simulink model "sei"  (Simulink 6.2)
settings: Solver=ode45  StartTime=0.0  StopTime=10.0  RelTol=1e-3
libraries: dsparch4 x287, cdsEpicsOut x108, cdsEpicsIn x18, cdsRms x18, Matrix8x x15, cdsSwitch1 x12, cdsProduct x9, Matrix88 x9, cdsSwitch x6, cdsSubtract8 x3, cdsRampSwitch x3, cdsSWD1 x3
(part 2 of 6)

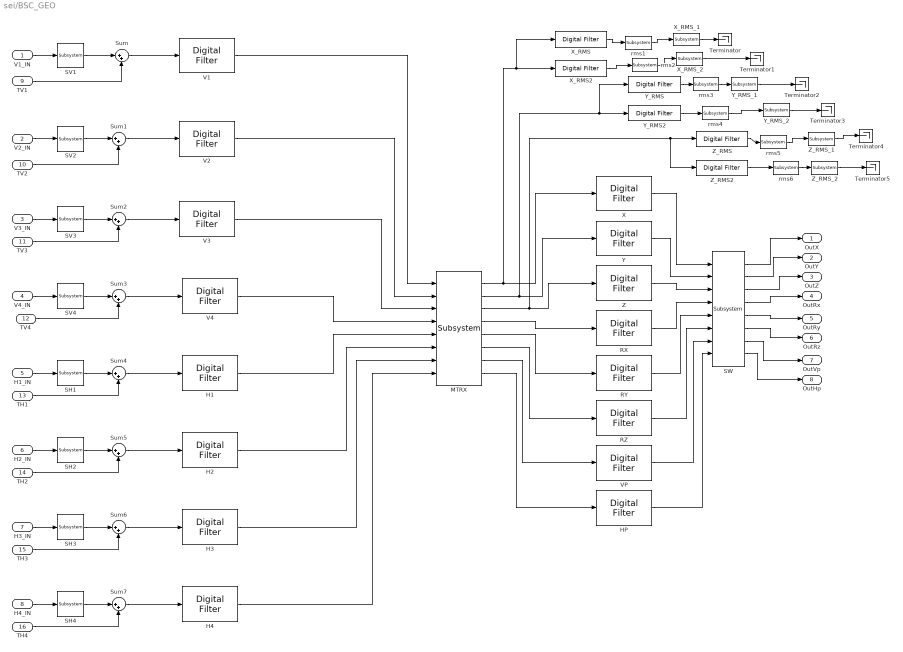
== system sei/BSC_GEO ==
  V1_IN : Inport  Port=1  LatchInput=off
  V2_IN : Inport  Port=2  LatchInput=off
  V3_IN : Inport  Port=3  LatchInput=off
  V4_IN : Inport  Port=4  LatchInput=off
  H1_IN : Inport  Port=5  LatchInput=off
  H2_IN : Inport  Port=6  LatchInput=off
  H3_IN : Inport  Port=7  LatchInput=off
  H4_IN : Inport  Port=8  LatchInput=off
  TV1 : Inport  Port=9  LatchInput=off
  TV2 : Inport  Port=10  LatchInput=off
  TV3 : Inport  Port=11  LatchInput=off
  TV4 : Inport  Port=12  LatchInput=off
  TH1 : Inport  Port=13  LatchInput=off
  TH2 : Inport  Port=14  LatchInput=off
  TH3 : Inport  Port=15  LatchInput=off
  TH4 : Inport  Port=16  LatchInput=off
  H1 : dsparch4/Digital Filter  DialogController=dspDDGCreate  DialogControllerArgs=DataTag26  TypePopup=IIR (poles & zeros)  IIRFiltStruct=Direct form II transposed  AllPoleFiltStruct=Direct form  FIRFiltStruct=Direct form  CoeffSource=Specify via dialog  NumCoeffs=[1 2]  DenCoeffs=[1 0.1]  BiQuadCoeffs=[1 0.3 0.4 1 0.1 0.2]  LatticeCoeffs=[0.2 0.4]  denIgnore=on  FiltPerSampPopup=One filter per frame  IC=0  ICnum=0  ICden=0  roundingMode=Floor  overflowMode=off  ScaleValues=1  scaleValueFracLength=14  stageInFracLength=15  stageOutFracLength=15
  H2 : dsparch4/Digital Filter  DialogController=dspDDGCreate  DialogControllerArgs=DataTag27  TypePopup=IIR (poles & zeros)  IIRFiltStruct=Direct form II transposed  AllPoleFiltStruct=Direct form  FIRFiltStruct=Direct form  CoeffSource=Specify via dialog  NumCoeffs=[1 2]  DenCoeffs=[1 0.1]  BiQuadCoeffs=[1 0.3 0.4 1 0.1 0.2]  LatticeCoeffs=[0.2 0.4]  denIgnore=on  FiltPerSampPopup=One filter per frame  IC=0  ICnum=0  ICden=0  roundingMode=Floor  overflowMode=off  ScaleValues=1  scaleValueFracLength=14  stageInFracLength=15  stageOutFracLength=15
  H3 : dsparch4/Digital Filter  DialogController=dspDDGCreate  DialogControllerArgs=DataTag28  TypePopup=IIR (poles & zeros)  IIRFiltStruct=Direct form II transposed  AllPoleFiltStruct=Direct form  FIRFiltStruct=Direct form  CoeffSource=Specify via dialog  NumCoeffs=[1 2]  DenCoeffs=[1 0.1]  BiQuadCoeffs=[1 0.3 0.4 1 0.1 0.2]  LatticeCoeffs=[0.2 0.4]  denIgnore=on  FiltPerSampPopup=One filter per frame  IC=0  ICnum=0  ICden=0  roundingMode=Floor  overflowMode=off  ScaleValues=1  scaleValueFracLength=14  stageInFracLength=15  stageOutFracLength=15
  H4 : dsparch4/Digital Filter  DialogController=dspDDGCreate  DialogControllerArgs=DataTag29  TypePopup=IIR (poles & zeros)  IIRFiltStruct=Direct form II transposed  AllPoleFiltStruct=Direct form  FIRFiltStruct=Direct form  CoeffSource=Specify via dialog  NumCoeffs=[1 2]  DenCoeffs=[1 0.1]  BiQuadCoeffs=[1 0.3 0.4 1 0.1 0.2]  LatticeCoeffs=[0.2 0.4]  denIgnore=on  FiltPerSampPopup=One filter per frame  IC=0  ICnum=0  ICden=0  roundingMode=Floor  overflowMode=off  ScaleValues=1  scaleValueFracLength=14  stageInFracLength=15  stageOutFracLength=15
  HP : dsparch4/Digital Filter  DialogController=dspDDGCreate  DialogControllerArgs=DataTag30  TypePopup=IIR (poles & zeros)  IIRFiltStruct=Direct form II transposed  AllPoleFiltStruct=Direct form  FIRFiltStruct=Direct form  CoeffSource=Specify via dialog  NumCoeffs=[1 2]  DenCoeffs=[1 0.1]  BiQuadCoeffs=[1 0.3 0.4 1 0.1 0.2]  LatticeCoeffs=[0.2 0.4]  denIgnore=on  FiltPerSampPopup=One filter per frame  IC=0  ICnum=0  ICden=0  roundingMode=Floor  overflowMode=off  ScaleValues=1  scaleValueFracLength=14  stageInFracLength=15  stageOutFracLength=15
  MTRX : Matrix8x/Subsystem
  RX : dsparch4/Digital Filter  DialogController=dspDDGCreate  DialogControllerArgs=DataTag31  TypePopup=IIR (poles & zeros)  IIRFiltStruct=Direct form II transposed  AllPoleFiltStruct=Direct form  FIRFiltStruct=Direct form  CoeffSource=Specify via dialog  NumCoeffs=[1 2]  DenCoeffs=[1 0.1]  BiQuadCoeffs=[1 0.3 0.4 1 0.1 0.2]  LatticeCoeffs=[0.2 0.4]  denIgnore=on  FiltPerSampPopup=One filter per frame  IC=0  ICnum=0  ICden=0  roundingMode=Floor  overflowMode=off  ScaleValues=1  scaleValueFracLength=14  stageInFracLength=15  stageOutFracLength=15
  RY : dsparch4/Digital Filter  DialogController=dspDDGCreate  DialogControllerArgs=DataTag32  TypePopup=IIR (poles & zeros)  IIRFiltStruct=Direct form II transposed  AllPoleFiltStruct=Direct form  FIRFiltStruct=Direct form  CoeffSource=Specify via dialog  NumCoeffs=[1 2]  DenCoeffs=[1 0.1]  BiQuadCoeffs=[1 0.3 0.4 1 0.1 0.2]  LatticeCoeffs=[0.2 0.4]  denIgnore=on  FiltPerSampPopup=One filter per frame  IC=0  ICnum=0  ICden=0  roundingMode=Floor  overflowMode=off  ScaleValues=1  scaleValueFracLength=14  stageInFracLength=15  stageOutFracLength=15
  RZ : dsparch4/Digital Filter  DialogController=dspDDGCreate  DialogControllerArgs=DataTag33  TypePopup=IIR (poles & zeros)  IIRFiltStruct=Direct form II transposed  AllPoleFiltStruct=Direct form  FIRFiltStruct=Direct form  CoeffSource=Specify via dialog  NumCoeffs=[1 2]  DenCoeffs=[1 0.1]  BiQuadCoeffs=[1 0.3 0.4 1 0.1 0.2]  LatticeCoeffs=[0.2 0.4]  denIgnore=on  FiltPerSampPopup=One filter per frame  IC=0  ICnum=0  ICden=0  roundingMode=Floor  overflowMode=off  ScaleValues=1  scaleValueFracLength=14  stageInFracLength=15  stageOutFracLength=15
  SH{1..4} (4 alike) : cdsEpicsOut/Subsystem
  SV{1..4} (4 alike) : cdsEpicsOut/Subsystem
  SW : cdsSwitch/Subsystem
  Sum{,1..7} (8 alike) : Sum  Inputs=|++
  Terminator{,1..5} (6 alike) : Terminator
  V1 : dsparch4/Digital Filter  DialogController=dspDDGCreate  DialogControllerArgs=DataTag34  TypePopup=IIR (poles & zeros)  IIRFiltStruct=Direct form II transposed  AllPoleFiltStruct=Direct form  FIRFiltStruct=Direct form  CoeffSource=Specify via dialog  NumCoeffs=[1 2]  DenCoeffs=[1 0.1]  BiQuadCoeffs=[1 0.3 0.4 1 0.1 0.2]  LatticeCoeffs=[0.2 0.4]  denIgnore=on  FiltPerSampPopup=One filter per frame  IC=0  ICnum=0  ICden=0  roundingMode=Floor  overflowMode=off  ScaleValues=1  scaleValueFracLength=14  stageInFracLength=15  stageOutFracLength=15
  V2 : dsparch4/Digital Filter  DialogController=dspDDGCreate  DialogControllerArgs=DataTag35  TypePopup=IIR (poles & zeros)  IIRFiltStruct=Direct form II transposed  AllPoleFiltStruct=Direct form  FIRFiltStruct=Direct form  CoeffSource=Specify via dialog  NumCoeffs=[1 2]  DenCoeffs=[1 0.1]  BiQuadCoeffs=[1 0.3 0.4 1 0.1 0.2]  LatticeCoeffs=[0.2 0.4]  denIgnore=on  FiltPerSampPopup=One filter per frame  IC=0  ICnum=0  ICden=0  roundingMode=Floor  overflowMode=off  ScaleValues=1  scaleValueFracLength=14  stageInFracLength=15  stageOutFracLength=15
  V3 : dsparch4/Digital Filter  DialogController=dspDDGCreate  DialogControllerArgs=DataTag36  TypePopup=IIR (poles & zeros)  IIRFiltStruct=Direct form II transposed  AllPoleFiltStruct=Direct form  FIRFiltStruct=Direct form  CoeffSource=Specify via dialog  NumCoeffs=[1 2]  DenCoeffs=[1 0.1]  BiQuadCoeffs=[1 0.3 0.4 1 0.1 0.2]  LatticeCoeffs=[0.2 0.4]  denIgnore=on  FiltPerSampPopup=One filter per frame  IC=0  ICnum=0  ICden=0  roundingMode=Floor  overflowMode=off  ScaleValues=1  scaleValueFracLength=14  stageInFracLength=15  stageOutFracLength=15
  V4 : dsparch4/Digital Filter  DialogController=dspDDGCreate  DialogControllerArgs=DataTag37  TypePopup=IIR (poles & zeros)  IIRFiltStruct=Direct form II transposed  AllPoleFiltStruct=Direct form  FIRFiltStruct=Direct form  CoeffSource=Specify via dialog  NumCoeffs=[1 2]  DenCoeffs=[1 0.1]  BiQuadCoeffs=[1 0.3 0.4 1 0.1 0.2]  LatticeCoeffs=[0.2 0.4]  denIgnore=on  FiltPerSampPopup=One filter per frame  IC=0  ICnum=0  ICden=0  roundingMode=Floor  overflowMode=off  ScaleValues=1  scaleValueFracLength=14  stageInFracLength=15  stageOutFracLength=15
  VP : dsparch4/Digital Filter  DialogController=dspDDGCreate  DialogControllerArgs=DataTag38  TypePopup=IIR (poles & zeros)  IIRFiltStruct=Direct form II transposed  AllPoleFiltStruct=Direct form  FIRFiltStruct=Direct form  CoeffSource=Specify via dialog  NumCoeffs=[1 2]  DenCoeffs=[1 0.1]  BiQuadCoeffs=[1 0.3 0.4 1 0.1 0.2]  LatticeCoeffs=[0.2 0.4]  denIgnore=on  FiltPerSampPopup=One filter per frame  IC=0  ICnum=0  ICden=0  roundingMode=Floor  overflowMode=off  ScaleValues=1  scaleValueFracLength=14  stageInFracLength=15  stageOutFracLength=15
  X : dsparch4/Digital Filter  DialogController=dspDDGCreate  DialogControllerArgs=DataTag39  TypePopup=IIR (poles & zeros)  IIRFiltStruct=Direct form II transposed  AllPoleFiltStruct=Direct form  FIRFiltStruct=Direct form  CoeffSource=Specify via dialog  NumCoeffs=[1 2]  DenCoeffs=[1 0.1]  BiQuadCoeffs=[1 0.3 0.4 1 0.1 0.2]  LatticeCoeffs=[0.2 0.4]  denIgnore=on  FiltPerSampPopup=One filter per frame  IC=0  ICnum=0  ICden=0  roundingMode=Floor  overflowMode=off  ScaleValues=1  scaleValueFracLength=14  stageInFracLength=15  stageOutFracLength=15
  X_RMS : dsparch4/Digital Filter  DialogController=dspDDGCreate  DialogControllerArgs=DataTag40  TypePopup=IIR (poles & zeros)  IIRFiltStruct=Direct form II transposed  AllPoleFiltStruct=Direct form  FIRFiltStruct=Direct form  CoeffSource=Specify via dialog  NumCoeffs=[1 2]  DenCoeffs=[1 0.1]  BiQuadCoeffs=[1 0.3 0.4 1 0.1 0.2]  LatticeCoeffs=[0.2 0.4]  denIgnore=on  FiltPerSampPopup=One filter per frame  IC=0  ICnum=0  ICden=0  roundingMode=Floor  overflowMode=off  ScaleValues=1  scaleValueFracLength=14  stageInFracLength=15  stageOutFracLength=15
  X_RMS2 : dsparch4/Digital Filter  DialogController=dspDDGCreate  DialogControllerArgs=DataTag41  TypePopup=IIR (poles & zeros)  IIRFiltStruct=Direct form II transposed  AllPoleFiltStruct=Direct form  FIRFiltStruct=Direct form  CoeffSource=Specify via dialog  NumCoeffs=[1 2]  DenCoeffs=[1 0.1]  BiQuadCoeffs=[1 0.3 0.4 1 0.1 0.2]  LatticeCoeffs=[0.2 0.4]  denIgnore=on  FiltPerSampPopup=One filter per frame  IC=0  ICnum=0  ICden=0  roundingMode=Floor  overflowMode=off  ScaleValues=1  scaleValueFracLength=14  stageInFracLength=15  stageOutFracLength=15
  X_RMS_1 : cdsEpicsOut/Subsystem
  X_RMS_2 : cdsEpicsOut/Subsystem
  Y : dsparch4/Digital Filter  DialogController=dspDDGCreate  DialogControllerArgs=DataTag42  TypePopup=IIR (poles & zeros)  IIRFiltStruct=Direct form II transposed  AllPoleFiltStruct=Direct form  FIRFiltStruct=Direct form  CoeffSource=Specify via dialog  NumCoeffs=[1 2]  DenCoeffs=[1 0.1]  BiQuadCoeffs=[1 0.3 0.4 1 0.1 0.2]  LatticeCoeffs=[0.2 0.4]  denIgnore=on  FiltPerSampPopup=One filter per frame  IC=0  ICnum=0  ICden=0  roundingMode=Floor  overflowMode=off  ScaleValues=1  scaleValueFracLength=14  stageInFracLength=15  stageOutFracLength=15
  Y_RMS : dsparch4/Digital Filter  DialogController=dspDDGCreate  DialogControllerArgs=DataTag43  TypePopup=IIR (poles & zeros)  IIRFiltStruct=Direct form II transposed  AllPoleFiltStruct=Direct form  FIRFiltStruct=Direct form  CoeffSource=Specify via dialog  NumCoeffs=[1 2]  DenCoeffs=[1 0.1]  BiQuadCoeffs=[1 0.3 0.4 1 0.1 0.2]  LatticeCoeffs=[0.2 0.4]  denIgnore=on  FiltPerSampPopup=One filter per frame  IC=0  ICnum=0  ICden=0  roundingMode=Floor  overflowMode=off  ScaleValues=1  scaleValueFracLength=14  stageInFracLength=15  stageOutFracLength=15
  Y_RMS2 : dsparch4/Digital Filter  DialogController=dspDDGCreate  DialogControllerArgs=DataTag44  TypePopup=IIR (poles & zeros)  IIRFiltStruct=Direct form II transposed  AllPoleFiltStruct=Direct form  FIRFiltStruct=Direct form  CoeffSource=Specify via dialog  NumCoeffs=[1 2]  DenCoeffs=[1 0.1]  BiQuadCoeffs=[1 0.3 0.4 1 0.1 0.2]  LatticeCoeffs=[0.2 0.4]  denIgnore=on  FiltPerSampPopup=One filter per frame  IC=0  ICnum=0  ICden=0  roundingMode=Floor  overflowMode=off  ScaleValues=1  scaleValueFracLength=14  stageInFracLength=15  stageOutFracLength=15
  Y_RMS_1 : cdsEpicsOut/Subsystem
  Y_RMS_2 : cdsEpicsOut/Subsystem
  Z : dsparch4/Digital Filter  DialogController=dspDDGCreate  DialogControllerArgs=DataTag45  TypePopup=IIR (poles & zeros)  IIRFiltStruct=Direct form II transposed  AllPoleFiltStruct=Direct form  FIRFiltStruct=Direct form  CoeffSource=Specify via dialog  NumCoeffs=[1 2]  DenCoeffs=[1 0.1]  BiQuadCoeffs=[1 0.3 0.4 1 0.1 0.2]  LatticeCoeffs=[0.2 0.4]  denIgnore=on  FiltPerSampPopup=One filter per frame  IC=0  ICnum=0  ICden=0  roundingMode=Floor  overflowMode=off  ScaleValues=1  scaleValueFracLength=14  stageInFracLength=15  stageOutFracLength=15
  Z_RMS : dsparch4/Digital Filter  DialogController=dspDDGCreate  DialogControllerArgs=DataTag46  TypePopup=IIR (poles & zeros)  IIRFiltStruct=Direct form II transposed  AllPoleFiltStruct=Direct form  FIRFiltStruct=Direct form  CoeffSource=Specify via dialog  NumCoeffs=[1 2]  DenCoeffs=[1 0.1]  BiQuadCoeffs=[1 0.3 0.4 1 0.1 0.2]  LatticeCoeffs=[0.2 0.4]  denIgnore=on  FiltPerSampPopup=One filter per frame  IC=0  ICnum=0  ICden=0  roundingMode=Floor  overflowMode=off  ScaleValues=1  scaleValueFracLength=14  stageInFracLength=15  stageOutFracLength=15
  Z_RMS2 : dsparch4/Digital Filter  DialogController=dspDDGCreate  DialogControllerArgs=DataTag47  TypePopup=IIR (poles & zeros)  IIRFiltStruct=Direct form II transposed  AllPoleFiltStruct=Direct form  FIRFiltStruct=Direct form  CoeffSource=Specify via dialog  NumCoeffs=[1 2]  DenCoeffs=[1 0.1]  BiQuadCoeffs=[1 0.3 0.4 1 0.1 0.2]  LatticeCoeffs=[0.2 0.4]  denIgnore=on  FiltPerSampPopup=One filter per frame  IC=0  ICnum=0  ICden=0  roundingMode=Floor  overflowMode=off  ScaleValues=1  scaleValueFracLength=14  stageInFracLength=15  stageOutFracLength=15
  Z_RMS_1 : cdsEpicsOut/Subsystem
  Z_RMS_2 : cdsEpicsOut/Subsystem
  rms{1..6} (6 alike) : cdsRms/Subsystem
  OutX : Outport
  OutY : Outport  Port=2
  OutZ : Outport  Port=3
  OutRx : Outport  Port=4
  OutRy : Outport  Port=5
  OutRz : Outport  Port=6
  OutVp : Outport  Port=7
  OutHp : Outport  Port=8
  wires:
  H2_IN/1 -> SH2/1
  H3_IN/1 -> SH3/1
  H4_IN/1 -> SH4/1
  MTRX/1 -> X/1, X_RMS2/1, X_RMS/1
  MTRX/2 -> Y/1, Y_RMS2/1, Y_RMS/1
  MTRX/3 -> Z/1, Z_RMS/1, Z_RMS2/1
  MTRX/6 -> RZ/1
  MTRX/7 -> VP/1
  MTRX/8 -> HP/1
  X/1 -> SW/1
  Y/1 -> SW/2
  Z/1 -> SW/3
  RX/1 -> SW/4
  RY/1 -> SW/5
  RZ/1 -> SW/6
  VP/1 -> SW/7
  HP/1 -> SW/8
  MTRX/4 -> RX/1
  MTRX/5 -> RY/1
  SW/1 -> OutX/1
  SW/2 -> OutY/1
  SW/3 -> OutZ/1
  SW/4 -> OutRx/1
  SW/5 -> OutRy/1
  SW/6 -> OutRz/1
  SW/7 -> OutVp/1
  SW/8 -> OutHp/1
  V1/1 -> MTRX/1
  V2/1 -> MTRX/2
  V3/1 -> MTRX/3
  V4/1 -> MTRX/4
  H1/1 -> MTRX/5
  H2/1 -> MTRX/6
  H3/1 -> MTRX/7
  H4/1 -> MTRX/8
  H1_IN/1 -> SH1/1
  V4_IN/1 -> SV4/1
  V3_IN/1 -> SV3/1
  V2_IN/1 -> SV2/1
  V1_IN/1 -> SV1/1
  SV1/1 -> Sum/1
  SV2/1 -> Sum1/1
  SV3/1 -> Sum2/1
  SV4/1 -> Sum3/1
  SH1/1 -> Sum4/1
  SH2/1 -> Sum5/1
  SH3/1 -> Sum6/1
  SH4/1 -> Sum7/1
  TV1/1 -> Sum/2
  TV2/1 -> Sum1/2
  TV3/1 -> Sum2/2
  TV4/1 -> Sum3/2
  TH1/1 -> Sum4/2
  TH2/1 -> Sum5/2
  TH3/1 -> Sum6/2
  TH4/1 -> Sum7/2
  Sum3/1 -> V4/1
  Sum4/1 -> H1/1
  Sum5/1 -> H2/1
  Sum6/1 -> H3/1
  Sum7/1 -> H4/1
  Sum/1 -> V1/1
  Sum1/1 -> V2/1
  Sum2/1 -> V3/1
  X_RMS_1/1 -> Terminator/1
  X_RMS_2/1 -> Terminator1/1
  Y_RMS_2/1 -> Terminator3/1
  Y_RMS_1/1 -> Terminator2/1
  Z_RMS_1/1 -> Terminator4/1
  Z_RMS_2/1 -> Terminator5/1
  X_RMS2/1 -> rms2/1
  X_RMS/1 -> rms1/1
  rms1/1 -> X_RMS_1/1
  rms2/1 -> X_RMS_2/1
  Y_RMS2/1 -> rms4/1
  Y_RMS/1 -> rms3/1
  rms3/1 -> Y_RMS_1/1
  rms4/1 -> Y_RMS_2/1
  Z_RMS2/1 -> rms6/1
  rms6/1 -> Z_RMS_2/1
  Z_RMS/1 -> rms5/1
  rms5/1 -> Z_RMS_1/1

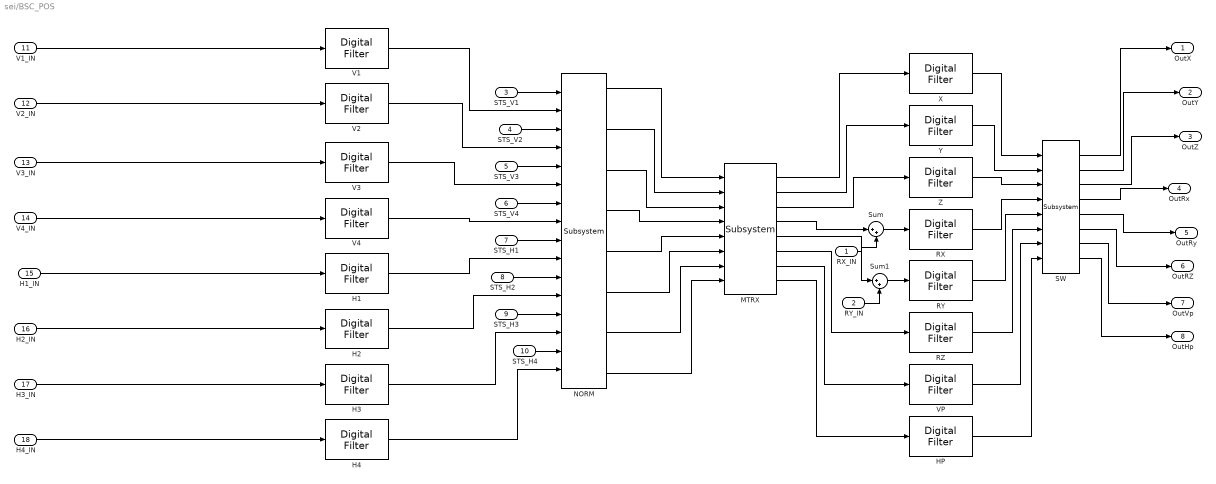
== system sei/BSC_POS ==
  RX_IN : Inport  Port=1  LatchInput=off
  RY_IN : Inport  Port=2  LatchInput=off
  STS_V1 : Inport  Port=3  LatchInput=off
  STS_V2 : Inport  Port=4  LatchInput=off
  STS_V3 : Inport  Port=5  LatchInput=off
  STS_V4 : Inport  Port=6  LatchInput=off
  STS_H1 : Inport  Port=7  LatchInput=off
  STS_H2 : Inport  Port=8  LatchInput=off
  STS_H3 : Inport  Port=9  LatchInput=off
  STS_H4 : Inport  Port=10  LatchInput=off
  V1_IN : Inport  Port=11  LatchInput=off
  V2_IN : Inport  Port=12  LatchInput=off
  V3_IN : Inport  Port=13  LatchInput=off
  V4_IN : Inport  Port=14  LatchInput=off
  H1_IN : Inport  Port=15  LatchInput=off
  H2_IN : Inport  Port=16  LatchInput=off
  H3_IN : Inport  Port=17  LatchInput=off
  H4_IN : Inport  Port=18  LatchInput=off
  H1 : dsparch4/Digital Filter  DialogController=dspDDGCreate  DialogControllerArgs=DataTag48  TypePopup=IIR (poles & zeros)  IIRFiltStruct=Direct form II transposed  AllPoleFiltStruct=Direct form  FIRFiltStruct=Direct form  CoeffSource=Specify via dialog  NumCoeffs=[1 2]  DenCoeffs=[1 0.1]  BiQuadCoeffs=[1 0.3 0.4 1 0.1 0.2]  LatticeCoeffs=[0.2 0.4]  denIgnore=on  FiltPerSampPopup=One filter per frame  IC=0  ICnum=0  ICden=0  roundingMode=Floor  overflowMode=off  ScaleValues=1  scaleValueFracLength=14  stageInFracLength=15  stageOutFracLength=15
  H2 : dsparch4/Digital Filter  DialogController=dspDDGCreate  DialogControllerArgs=DataTag49  TypePopup=IIR (poles & zeros)  IIRFiltStruct=Direct form II transposed  AllPoleFiltStruct=Direct form  FIRFiltStruct=Direct form  CoeffSource=Specify via dialog  NumCoeffs=[1 2]  DenCoeffs=[1 0.1]  BiQuadCoeffs=[1 0.3 0.4 1 0.1 0.2]  LatticeCoeffs=[0.2 0.4]  denIgnore=on  FiltPerSampPopup=One filter per frame  IC=0  ICnum=0  ICden=0  roundingMode=Floor  overflowMode=off  ScaleValues=1  scaleValueFracLength=14  stageInFracLength=15  stageOutFracLength=15
  H3 : dsparch4/Digital Filter  DialogController=dspDDGCreate  DialogControllerArgs=DataTag50  TypePopup=IIR (poles & zeros)  IIRFiltStruct=Direct form II transposed  AllPoleFiltStruct=Direct form  FIRFiltStruct=Direct form  CoeffSource=Specify via dialog  NumCoeffs=[1 2]  DenCoeffs=[1 0.1]  BiQuadCoeffs=[1 0.3 0.4 1 0.1 0.2]  LatticeCoeffs=[0.2 0.4]  denIgnore=on  FiltPerSampPopup=One filter per frame  IC=0  ICnum=0  ICden=0  roundingMode=Floor  overflowMode=off  ScaleValues=1  scaleValueFracLength=14  stageInFracLength=15  stageOutFracLength=15
  H4 : dsparch4/Digital Filter  DialogController=dspDDGCreate  DialogControllerArgs=DataTag51  TypePopup=IIR (poles & zeros)  IIRFiltStruct=Direct form II transposed  AllPoleFiltStruct=Direct form  FIRFiltStruct=Direct form  CoeffSource=Specify via dialog  NumCoeffs=[1 2]  DenCoeffs=[1 0.1]  BiQuadCoeffs=[1 0.3 0.4 1 0.1 0.2]  LatticeCoeffs=[0.2 0.4]  denIgnore=on  FiltPerSampPopup=One filter per frame  IC=0  ICnum=0  ICden=0  roundingMode=Floor  overflowMode=off  ScaleValues=1  scaleValueFracLength=14  stageInFracLength=15  stageOutFracLength=15
  HP : dsparch4/Digital Filter  DialogController=dspDDGCreate  DialogControllerArgs=DataTag52  TypePopup=IIR (poles & zeros)  IIRFiltStruct=Direct form II transposed  AllPoleFiltStruct=Direct form  FIRFiltStruct=Direct form  CoeffSource=Specify via dialog  NumCoeffs=[1 2]  DenCoeffs=[1 0.1]  BiQuadCoeffs=[1 0.3 0.4 1 0.1 0.2]  LatticeCoeffs=[0.2 0.4]  denIgnore=on  FiltPerSampPopup=One filter per frame  IC=0  ICnum=0  ICden=0  roundingMode=Floor  overflowMode=off  ScaleValues=1  scaleValueFracLength=14  stageInFracLength=15  stageOutFracLength=15
  MTRX : Matrix8x/Subsystem
  NORM : cdsSubtract8/Subsystem
  RX : dsparch4/Digital Filter  DialogController=dspDDGCreate  DialogControllerArgs=DataTag53  TypePopup=IIR (poles & zeros)  IIRFiltStruct=Direct form II transposed  AllPoleFiltStruct=Direct form  FIRFiltStruct=Direct form  CoeffSource=Specify via dialog  NumCoeffs=[1 2]  DenCoeffs=[1 0.1]  BiQuadCoeffs=[1 0.3 0.4 1 0.1 0.2]  LatticeCoeffs=[0.2 0.4]  denIgnore=on  FiltPerSampPopup=One filter per frame  IC=0  ICnum=0  ICden=0  roundingMode=Floor  overflowMode=off  ScaleValues=1  scaleValueFracLength=14  stageInFracLength=15  stageOutFracLength=15
  RY : dsparch4/Digital Filter  DialogController=dspDDGCreate  DialogControllerArgs=DataTag54  TypePopup=IIR (poles & zeros)  IIRFiltStruct=Direct form II transposed  AllPoleFiltStruct=Direct form  FIRFiltStruct=Direct form  CoeffSource=Specify via dialog  NumCoeffs=[1 2]  DenCoeffs=[1 0.1]  BiQuadCoeffs=[1 0.3 0.4 1 0.1 0.2]  LatticeCoeffs=[0.2 0.4]  denIgnore=on  FiltPerSampPopup=One filter per frame  IC=0  ICnum=0  ICden=0  roundingMode=Floor  overflowMode=off  ScaleValues=1  scaleValueFracLength=14  stageInFracLength=15  stageOutFracLength=15
  RZ : dsparch4/Digital Filter  DialogController=dspDDGCreate  DialogControllerArgs=DataTag55  TypePopup=IIR (poles & zeros)  IIRFiltStruct=Direct form II transposed  AllPoleFiltStruct=Direct form  FIRFiltStruct=Direct form  CoeffSource=Specify via dialog  NumCoeffs=[1 2]  DenCoeffs=[1 0.1]  BiQuadCoeffs=[1 0.3 0.4 1 0.1 0.2]  LatticeCoeffs=[0.2 0.4]  denIgnore=on  FiltPerSampPopup=One filter per frame  IC=0  ICnum=0  ICden=0  roundingMode=Floor  overflowMode=off  ScaleValues=1  scaleValueFracLength=14  stageInFracLength=15  stageOutFracLength=15
  SW : cdsSwitch/Subsystem
  Sum : Sum  Inputs=|++
  Sum1 : Sum  Inputs=|++
  V1 : dsparch4/Digital Filter  DialogController=dspDDGCreate  DialogControllerArgs=DataTag56  TypePopup=IIR (poles & zeros)  IIRFiltStruct=Direct form II transposed  AllPoleFiltStruct=Direct form  FIRFiltStruct=Direct form  CoeffSource=Specify via dialog  NumCoeffs=[1 2]  DenCoeffs=[1 0.1]  BiQuadCoeffs=[1 0.3 0.4 1 0.1 0.2]  LatticeCoeffs=[0.2 0.4]  denIgnore=on  FiltPerSampPopup=One filter per frame  IC=0  ICnum=0  ICden=0  roundingMode=Floor  overflowMode=off  ScaleValues=1  scaleValueFracLength=14  stageInFracLength=15  stageOutFracLength=15
  V2 : dsparch4/Digital Filter  DialogController=dspDDGCreate  DialogControllerArgs=DataTag57  TypePopup=IIR (poles & zeros)  IIRFiltStruct=Direct form II transposed  AllPoleFiltStruct=Direct form  FIRFiltStruct=Direct form  CoeffSource=Specify via dialog  NumCoeffs=[1 2]  DenCoeffs=[1 0.1]  BiQuadCoeffs=[1 0.3 0.4 1 0.1 0.2]  LatticeCoeffs=[0.2 0.4]  denIgnore=on  FiltPerSampPopup=One filter per frame  IC=0  ICnum=0  ICden=0  roundingMode=Floor  overflowMode=off  ScaleValues=1  scaleValueFracLength=14  stageInFracLength=15  stageOutFracLength=15
  V3 : dsparch4/Digital Filter  DialogController=dspDDGCreate  DialogControllerArgs=DataTag58  TypePopup=IIR (poles & zeros)  IIRFiltStruct=Direct form II transposed  AllPoleFiltStruct=Direct form  FIRFiltStruct=Direct form  CoeffSource=Specify via dialog  NumCoeffs=[1 2]  DenCoeffs=[1 0.1]  BiQuadCoeffs=[1 0.3 0.4 1 0.1 0.2]  LatticeCoeffs=[0.2 0.4]  denIgnore=on  FiltPerSampPopup=One filter per frame  IC=0  ICnum=0  ICden=0  roundingMode=Floor  overflowMode=off  ScaleValues=1  scaleValueFracLength=14  stageInFracLength=15  stageOutFracLength=15
  V4 : dsparch4/Digital Filter  DialogController=dspDDGCreate  DialogControllerArgs=DataTag59  TypePopup=IIR (poles & zeros)  IIRFiltStruct=Direct form II transposed  AllPoleFiltStruct=Direct form  FIRFiltStruct=Direct form  CoeffSource=Specify via dialog  NumCoeffs=[1 2]  DenCoeffs=[1 0.1]  BiQuadCoeffs=[1 0.3 0.4 1 0.1 0.2]  LatticeCoeffs=[0.2 0.4]  denIgnore=on  FiltPerSampPopup=One filter per frame  IC=0  ICnum=0  ICden=0  roundingMode=Floor  overflowMode=off  ScaleValues=1  scaleValueFracLength=14  stageInFracLength=15  stageOutFracLength=15
  VP : dsparch4/Digital Filter  DialogController=dspDDGCreate  DialogControllerArgs=DataTag60  TypePopup=IIR (poles & zeros)  IIRFiltStruct=Direct form II transposed  AllPoleFiltStruct=Direct form  FIRFiltStruct=Direct form  CoeffSource=Specify via dialog  NumCoeffs=[1 2]  DenCoeffs=[1 0.1]  BiQuadCoeffs=[1 0.3 0.4 1 0.1 0.2]  LatticeCoeffs=[0.2 0.4]  denIgnore=on  FiltPerSampPopup=One filter per frame  IC=0  ICnum=0  ICden=0  roundingMode=Floor  overflowMode=off  ScaleValues=1  scaleValueFracLength=14  stageInFracLength=15  stageOutFracLength=15
  X : dsparch4/Digital Filter  DialogController=dspDDGCreate  DialogControllerArgs=DataTag61  TypePopup=IIR (poles & zeros)  IIRFiltStruct=Direct form II transposed  AllPoleFiltStruct=Direct form  FIRFiltStruct=Direct form  CoeffSource=Specify via dialog  NumCoeffs=[1 2]  DenCoeffs=[1 0.1]  BiQuadCoeffs=[1 0.3 0.4 1 0.1 0.2]  LatticeCoeffs=[0.2 0.4]  denIgnore=on  FiltPerSampPopup=One filter per frame  IC=0  ICnum=0  ICden=0  roundingMode=Floor  overflowMode=off  ScaleValues=1  scaleValueFracLength=14  stageInFracLength=15  stageOutFracLength=15
  Y : dsparch4/Digital Filter  DialogController=dspDDGCreate  DialogControllerArgs=DataTag62  TypePopup=IIR (poles & zeros)  IIRFiltStruct=Direct form II transposed  AllPoleFiltStruct=Direct form  FIRFiltStruct=Direct form  CoeffSource=Specify via dialog  NumCoeffs=[1 2]  DenCoeffs=[1 0.1]  BiQuadCoeffs=[1 0.3 0.4 1 0.1 0.2]  LatticeCoeffs=[0.2 0.4]  denIgnore=on  FiltPerSampPopup=One filter per frame  IC=0  ICnum=0  ICden=0  roundingMode=Floor  overflowMode=off  ScaleValues=1  scaleValueFracLength=14  stageInFracLength=15  stageOutFracLength=15
  Z : dsparch4/Digital Filter  DialogController=dspDDGCreate  DialogControllerArgs=DataTag63  TypePopup=IIR (poles & zeros)  IIRFiltStruct=Direct form II transposed  AllPoleFiltStruct=Direct form  FIRFiltStruct=Direct form  CoeffSource=Specify via dialog  NumCoeffs=[1 2]  DenCoeffs=[1 0.1]  BiQuadCoeffs=[1 0.3 0.4 1 0.1 0.2]  LatticeCoeffs=[0.2 0.4]  denIgnore=on  FiltPerSampPopup=One filter per frame  IC=0  ICnum=0  ICden=0  roundingMode=Floor  overflowMode=off  ScaleValues=1  scaleValueFracLength=14  stageInFracLength=15  stageOutFracLength=15
  OutX : Outport
  OutY : Outport  Port=2
  OutZ : Outport  Port=3
  OutRx : Outport  Port=4
  OutRy : Outport  Port=5
  OutRZ : Outport  Port=6
  OutVp : Outport  Port=7
  OutHp : Outport  Port=8
  wires:
  V1_IN/1 -> V1/1
  V2_IN/1 -> V2/1
  V3_IN/1 -> V3/1
  V4_IN/1 -> V4/1
  H1_IN/1 -> H1/1
  H2_IN/1 -> H2/1
  H3_IN/1 -> H3/1
  H4_IN/1 -> H4/1
  V1/1 -> NORM/2
  V2/1 -> NORM/4
  V3/1 -> NORM/6
  V4/1 -> NORM/8
  H1/1 -> NORM/10
  H2/1 -> NORM/12
  H3/1 -> NORM/14
  H4/1 -> NORM/16
  STS_V1/1 -> NORM/1
  STS_V2/1 -> NORM/3
  STS_V3/1 -> NORM/5
  STS_V4/1 -> NORM/7
  STS_H1/1 -> NORM/9
  STS_H2/1 -> NORM/11
  STS_H3/1 -> NORM/13
  STS_H4/1 -> NORM/15
  MTRX/1 -> X/1
  MTRX/2 -> Y/1
  MTRX/3 -> Z/1
  MTRX/6 -> RZ/1
  MTRX/7 -> VP/1
  MTRX/8 -> HP/1
  Sum1/1 -> RY/1
  Sum/1 -> RX/1
  MTRX/4 -> Sum/1
  MTRX/5 -> Sum1/1
  X/1 -> SW/1
  Y/1 -> SW/2
  Z/1 -> SW/3
  RX/1 -> SW/4
  RY/1 -> SW/5
  RZ/1 -> SW/6
  VP/1 -> SW/7
  HP/1 -> SW/8
  RX_IN/1 -> Sum/2
  RY_IN/1 -> Sum1/2
  NORM/1 -> MTRX/1
  NORM/2 -> MTRX/2
  NORM/3 -> MTRX/3
  NORM/4 -> MTRX/4
  NORM/5 -> MTRX/5
  NORM/6 -> MTRX/6
  NORM/7 -> MTRX/7
  NORM/8 -> MTRX/8
  SW/1 -> OutX/1
  SW/2 -> OutY/1
  SW/3 -> OutZ/1
  SW/4 -> OutRx/1
  SW/5 -> OutRy/1
  SW/6 -> OutRZ/1
  SW/7 -> OutVp/1
  SW/8 -> OutHp/1

== system sei/BSC_SPARE ==
  In1 : Inport  Port=1  LatchInput=off
  In2 : Inport  Port=2  LatchInput=off
  In3 : Inport  Port=3  LatchInput=off
  In4 : Inport  Port=4  LatchInput=off
  In5 : Inport  Port=5  LatchInput=off
  FP1 : dsparch4/Digital Filter  DialogController=dspDDGCreate  DialogControllerArgs=DataTag64  TypePopup=IIR (poles & zeros)  IIRFiltStruct=Direct form II transposed  AllPoleFiltStruct=Direct form  FIRFiltStruct=Direct form  CoeffSource=Specify via dialog  NumCoeffs=[1 2]  DenCoeffs=[1 0.1]  BiQuadCoeffs=[1 0.3 0.4 1 0.1 0.2]  LatticeCoeffs=[0.2 0.4]  denIgnore=on  FiltPerSampPopup=One filter per frame  IC=0  ICnum=0  ICden=0  roundingMode=Floor  overflowMode=off  ScaleValues=1  scaleValueFracLength=14  stageInFracLength=15  stageOutFracLength=15
  FP2 : dsparch4/Digital Filter  DialogController=dspDDGCreate  DialogControllerArgs=DataTag65  TypePopup=IIR (poles & zeros)  IIRFiltStruct=Direct form II transposed  AllPoleFiltStruct=Direct form  FIRFiltStruct=Direct form  CoeffSource=Specify via dialog  NumCoeffs=[1 2]  DenCoeffs=[1 0.1]  BiQuadCoeffs=[1 0.3 0.4 1 0.1 0.2]  LatticeCoeffs=[0.2 0.4]  denIgnore=on  FiltPerSampPopup=One filter per frame  IC=0  ICnum=0  ICden=0  roundingMode=Floor  overflowMode=off  ScaleValues=1  scaleValueFracLength=14  stageInFracLength=15  stageOutFracLength=15
  RP1 : dsparch4/Digital Filter  DialogController=dspDDGCreate  DialogControllerArgs=DataTag66  TypePopup=IIR (poles & zeros)  IIRFiltStruct=Direct form II transposed  AllPoleFiltStruct=Direct form  FIRFiltStruct=Direct form  CoeffSource=Specify via dialog  NumCoeffs=[1 2]  DenCoeffs=[1 0.1]  BiQuadCoeffs=[1 0.3 0.4 1 0.1 0.2]  LatticeCoeffs=[0.2 0.4]  denIgnore=on  FiltPerSampPopup=One filter per frame  IC=0  ICnum=0  ICden=0  roundingMode=Floor  overflowMode=off  ScaleValues=1  scaleValueFracLength=14  stageInFracLength=15  stageOutFracLength=15
  RP2 : dsparch4/Digital Filter  DialogController=dspDDGCreate  DialogControllerArgs=DataTag67  TypePopup=IIR (poles & zeros)  IIRFiltStruct=Direct form II transposed  AllPoleFiltStruct=Direct form  FIRFiltStruct=Direct form  CoeffSource=Specify via dialog  NumCoeffs=[1 2]  DenCoeffs=[1 0.1]  BiQuadCoeffs=[1 0.3 0.4 1 0.1 0.2]  LatticeCoeffs=[0.2 0.4]  denIgnore=on  FiltPerSampPopup=One filter per frame  IC=0  ICnum=0  ICden=0  roundingMode=Floor  overflowMode=off  ScaleValues=1  scaleValueFracLength=14  stageInFracLength=15  stageOutFracLength=15
  RP3 : dsparch4/Digital Filter  DialogController=dspDDGCreate  DialogControllerArgs=DataTag68  TypePopup=IIR (poles & zeros)  IIRFiltStruct=Direct form II transposed  AllPoleFiltStruct=Direct form  FIRFiltStruct=Direct form  CoeffSource=Specify via dialog  NumCoeffs=[1 2]  DenCoeffs=[1 0.1]  BiQuadCoeffs=[1 0.3 0.4 1 0.1 0.2]  LatticeCoeffs=[0.2 0.4]  denIgnore=on  FiltPerSampPopup=One filter per frame  IC=0  ICnum=0  ICden=0  roundingMode=Floor  overflowMode=off  ScaleValues=1  scaleValueFracLength=14  stageInFracLength=15  stageOutFracLength=15
  Terminator{1..5} (5 alike) : Terminator
  wires:
  RP3/1 -> Terminator5/1
  RP2/1 -> Terminator4/1
  RP1/1 -> Terminator2/1
  FP2/1 -> Terminator1/1
  FP1/1 -> Terminator3/1
  In1/1 -> FP1/1
  In2/1 -> FP2/1
  In3/1 -> RP1/1
  In4/1 -> RP2/1
  In5/1 -> RP3/1

== system sei/BSC_STS ==
  X1 : Inport  Port=1  LatchInput=off
  Y1 : Inport  Port=2  LatchInput=off
  Z1 : Inport  Port=3  LatchInput=off
  X2 : Inport  Port=4  LatchInput=off
  Y2 : Inport  Port=5  LatchInput=off
  Z2 : Inport  Port=6  LatchInput=off
  FIR_X : Inport  Port=7  LatchInput=off
  FIR_Y : Inport  Port=8  LatchInput=off
  IN_MTRX : Matrix88/Subsystem
  MTRX : Matrix88/Subsystem
  RAMP_SW : cdsRampSwitch/Subsystem
  X : dsparch4/Digital Filter  DialogController=dspDDGCreate  DialogControllerArgs=DataTag69  TypePopup=IIR (poles & zeros)  IIRFiltStruct=Direct form II transposed  AllPoleFiltStruct=Direct form  FIRFiltStruct=Direct form  CoeffSource=Specify via dialog  NumCoeffs=[1 2]  DenCoeffs=[1 0.1]  BiQuadCoeffs=[1 0.3 0.4 1 0.1 0.2]  LatticeCoeffs=[0.2 0.4]  denIgnore=on  FiltPerSampPopup=One filter per frame  IC=0  ICnum=0  ICden=0  roundingMode=Floor  overflowMode=off  ScaleValues=1  scaleValueFracLength=14  stageInFracLength=15  stageOutFracLength=15
  X_RY : dsparch4/Digital Filter  DialogController=dspDDGCreate  DialogControllerArgs=DataTag70  TypePopup=IIR (poles & zeros)  IIRFiltStruct=Direct form II transposed  AllPoleFiltStruct=Direct form  FIRFiltStruct=Direct form  CoeffSource=Specify via dialog  NumCoeffs=[1 2]  DenCoeffs=[1 0.1]  BiQuadCoeffs=[1 0.3 0.4 1 0.1 0.2]  LatticeCoeffs=[0.2 0.4]  denIgnore=on  FiltPerSampPopup=One filter per frame  IC=0  ICnum=0  ICden=0  roundingMode=Floor  overflowMode=off  ScaleValues=1  scaleValueFracLength=14  stageInFracLength=15  stageOutFracLength=15
  Y : dsparch4/Digital Filter  DialogController=dspDDGCreate  DialogControllerArgs=DataTag71  TypePopup=IIR (poles & zeros)  IIRFiltStruct=Direct form II transposed  AllPoleFiltStruct=Direct form  FIRFiltStruct=Direct form  CoeffSource=Specify via dialog  NumCoeffs=[1 2]  DenCoeffs=[1 0.1]  BiQuadCoeffs=[1 0.3 0.4 1 0.1 0.2]  LatticeCoeffs=[0.2 0.4]  denIgnore=on  FiltPerSampPopup=One filter per frame  IC=0  ICnum=0  ICden=0  roundingMode=Floor  overflowMode=off  ScaleValues=1  scaleValueFracLength=14  stageInFracLength=15  stageOutFracLength=15
  Y_RX : dsparch4/Digital Filter  DialogController=dspDDGCreate  DialogControllerArgs=DataTag72  TypePopup=IIR (poles & zeros)  IIRFiltStruct=Direct form II transposed  AllPoleFiltStruct=Direct form  FIRFiltStruct=Direct form  CoeffSource=Specify via dialog  NumCoeffs=[1 2]  DenCoeffs=[1 0.1]  BiQuadCoeffs=[1 0.3 0.4 1 0.1 0.2]  LatticeCoeffs=[0.2 0.4]  denIgnore=on  FiltPerSampPopup=One filter per frame  IC=0  ICnum=0  ICden=0  roundingMode=Floor  overflowMode=off  ScaleValues=1  scaleValueFracLength=14  stageInFracLength=15  stageOutFracLength=15
  Z : dsparch4/Digital Filter  DialogController=dspDDGCreate  DialogControllerArgs=DataTag73  TypePopup=IIR (poles & zeros)  IIRFiltStruct=Direct form II transposed  AllPoleFiltStruct=Direct form  FIRFiltStruct=Direct form  CoeffSource=Specify via dialog  NumCoeffs=[1 2]  DenCoeffs=[1 0.1]  BiQuadCoeffs=[1 0.3 0.4 1 0.1 0.2]  LatticeCoeffs=[0.2 0.4]  denIgnore=on  FiltPerSampPopup=One filter per frame  IC=0  ICnum=0  ICden=0  roundingMode=Floor  overflowMode=off  ScaleValues=1  scaleValueFracLength=14  stageInFracLength=15  stageOutFracLength=15
  RX : Outport
  RY : Outport  Port=2
  V1 : Outport  Port=3
  V2 : Outport  Port=4
  V3 : Outport  Port=5
  V4 : Outport  Port=6
  H1 : Outport  Port=7
  H2 : Outport  Port=8
  H3 : Outport  Port=9
  H4 : Outport  Port=10
  WDX : Outport  Port=11
  WDY : Outport  Port=12
  WDZ : Outport  Port=13
  wires:
  IN_MTRX/2 -> Y/1, WDY/1
  IN_MTRX/1 -> X/1, WDX/1
  IN_MTRX/3 -> Z/1, WDZ/1
  Z/1 -> MTRX/3
  X_RY/1 -> RX/1
  Y_RX/1 -> RY/1
  X1/1 -> IN_MTRX/1
  MTRX/1 -> V1/1
  Y1/1 -> IN_MTRX/2
  MTRX/2 -> V2/1
  Z1/1 -> IN_MTRX/3
  MTRX/3 -> V3/1
  X2/1 -> IN_MTRX/4
  MTRX/4 -> V4/1
  Y2/1 -> IN_MTRX/5
  MTRX/5 -> H1/1
  Z2/1 -> IN_MTRX/6
  MTRX/6 -> H2/1
  MTRX/7 -> H3/1
  MTRX/8 -> H4/1
  X/1 -> RAMP_SW/1
  FIR_X/1 -> RAMP_SW/2
  Y/1 -> RAMP_SW/3
  FIR_Y/1 -> RAMP_SW/4
  RAMP_SW/2 -> MTRX/2, Y_RX/1
  RAMP_SW/1 -> MTRX/1, X_RY/1

== system sei/BSC_WD ==
  In1 : Inport  Port=1  LatchInput=off
  In2 : Inport  Port=2  LatchInput=off
  In3 : Inport  Port=3  LatchInput=off
  In4 : Inport  Port=4  LatchInput=off
  In5 : Inport  Port=5  LatchInput=off
  In6 : Inport  Port=6  LatchInput=off
  In7 : Inport  Port=7  LatchInput=off
  In8 : Inport  Port=8  LatchInput=off
  In9 : Inport  Port=9  LatchInput=off
  In10 : Inport  Port=10  LatchInput=off
  In11 : Inport  Port=11  LatchInput=off
  In12 : Inport  Port=12  LatchInput=off
  In13 : Inport  Port=13  LatchInput=off
  In14 : Inport  Port=14  LatchInput=off
  In15 : Inport  Port=15  LatchInput=off
  In16 : Inport  Port=16  LatchInput=off
  In17 : Inport  Port=17  LatchInput=off
  In18 : Inport  Port=18  LatchInput=off
  In19 : Inport  Port=19  LatchInput=off
  GEO_H1 : dsparch4/Digital Filter  DialogController=dspDDGCreate  DialogControllerArgs=DataTag74  TypePopup=IIR (poles & zeros)  IIRFiltStruct=Direct form II transposed  AllPoleFiltStruct=Direct form  FIRFiltStruct=Direct form  CoeffSource=Specify via dialog  NumCoeffs=[1 2]  DenCoeffs=[1 0.1]  BiQuadCoeffs=[1 0.3 0.4 1 0.1 0.2]  LatticeCoeffs=[0.2 0.4]  denIgnore=on  FiltPerSampPopup=One filter per frame  IC=0  ICnum=0  ICden=0  roundingMode=Floor  overflowMode=off  ScaleValues=1  scaleValueFracLength=14  stageInFracLength=15  stageOutFracLength=15
  GEO_H2 : dsparch4/Digital Filter  DialogController=dspDDGCreate  DialogControllerArgs=DataTag75  TypePopup=IIR (poles & zeros)  IIRFiltStruct=Direct form II transposed  AllPoleFiltStruct=Direct form  FIRFiltStruct=Direct form  CoeffSource=Specify via dialog  NumCoeffs=[1 2]  DenCoeffs=[1 0.1]  BiQuadCoeffs=[1 0.3 0.4 1 0.1 0.2]  LatticeCoeffs=[0.2 0.4]  denIgnore=on  FiltPerSampPopup=One filter per frame  IC=0  ICnum=0  ICden=0  roundingMode=Floor  overflowMode=off  ScaleValues=1  scaleValueFracLength=14  stageInFracLength=15  stageOutFracLength=15
  GEO_H3 : dsparch4/Digital Filter  DialogController=dspDDGCreate  DialogControllerArgs=DataTag76  TypePopup=IIR (poles & zeros)  IIRFiltStruct=Direct form II transposed  AllPoleFiltStruct=Direct form  FIRFiltStruct=Direct form  CoeffSource=Specify via dialog  NumCoeffs=[1 2]  DenCoeffs=[1 0.1]  BiQuadCoeffs=[1 0.3 0.4 1 0.1 0.2]  LatticeCoeffs=[0.2 0.4]  denIgnore=on  FiltPerSampPopup=One filter per frame  IC=0  ICnum=0  ICden=0  roundingMode=Floor  overflowMode=off  ScaleValues=1  scaleValueFracLength=14  stageInFracLength=15  stageOutFracLength=15
  GEO_H4 : dsparch4/Digital Filter  DialogController=dspDDGCreate  DialogControllerArgs=DataTag77  TypePopup=IIR (poles & zeros)  IIRFiltStruct=Direct form II transposed  AllPoleFiltStruct=Direct form  FIRFiltStruct=Direct form  CoeffSource=Specify via dialog  NumCoeffs=[1 2]  DenCoeffs=[1 0.1]  BiQuadCoeffs=[1 0.3 0.4 1 0.1 0.2]  LatticeCoeffs=[0.2 0.4]  denIgnore=on  FiltPerSampPopup=One filter per frame  IC=0  ICnum=0  ICden=0  roundingMode=Floor  overflowMode=off  ScaleValues=1  scaleValueFracLength=14  stageInFracLength=15  stageOutFracLength=15
  GEO_V1 : dsparch4/Digital Filter  DialogController=dspDDGCreate  DialogControllerArgs=DataTag78  TypePopup=IIR (poles & zeros)  IIRFiltStruct=Direct form II transposed  AllPoleFiltStruct=Direct form  FIRFiltStruct=Direct form  CoeffSource=Specify via dialog  NumCoeffs=[1 2]  DenCoeffs=[1 0.1]  BiQuadCoeffs=[1 0.3 0.4 1 0.1 0.2]  LatticeCoeffs=[0.2 0.4]  denIgnore=on  FiltPerSampPopup=One filter per frame  IC=0  ICnum=0  ICden=0  roundingMode=Floor  overflowMode=off  ScaleValues=1  scaleValueFracLength=14  stageInFracLength=15  stageOutFracLength=15
  GEO_V2 : dsparch4/Digital Filter  DialogController=dspDDGCreate  DialogControllerArgs=DataTag79  TypePopup=IIR (poles & zeros)  IIRFiltStruct=Direct form II transposed  AllPoleFiltStruct=Direct form  FIRFiltStruct=Direct form  CoeffSource=Specify via dialog  NumCoeffs=[1 2]  DenCoeffs=[1 0.1]  BiQuadCoeffs=[1 0.3 0.4 1 0.1 0.2]  LatticeCoeffs=[0.2 0.4]  denIgnore=on  FiltPerSampPopup=One filter per frame  IC=0  ICnum=0  ICden=0  roundingMode=Floor  overflowMode=off  ScaleValues=1  scaleValueFracLength=14  stageInFracLength=15  stageOutFracLength=15
  GEO_V3 : dsparch4/Digital Filter  DialogController=dspDDGCreate  DialogControllerArgs=DataTag80  TypePopup=IIR (poles & zeros)  IIRFiltStruct=Direct form II transposed  AllPoleFiltStruct=Direct form  FIRFiltStruct=Direct form  CoeffSource=Specify via dialog  NumCoeffs=[1 2]  DenCoeffs=[1 0.1]  BiQuadCoeffs=[1 0.3 0.4 1 0.1 0.2]  LatticeCoeffs=[0.2 0.4]  denIgnore=on  FiltPerSampPopup=One filter per frame  IC=0  ICnum=0  ICden=0  roundingMode=Floor  overflowMode=off  ScaleValues=1  scaleValueFracLength=14  stageInFracLength=15  stageOutFracLength=15
  GEO_V4 : dsparch4/Digital Filter  DialogController=dspDDGCreate  DialogControllerArgs=DataTag81  TypePopup=IIR (poles & zeros)  IIRFiltStruct=Direct form II transposed  AllPoleFiltStruct=Direct form  FIRFiltStruct=Direct form  CoeffSource=Specify via dialog  NumCoeffs=[1 2]  DenCoeffs=[1 0.1]  BiQuadCoeffs=[1 0.3 0.4 1 0.1 0.2]  LatticeCoeffs=[0.2 0.4]  denIgnore=on  FiltPerSampPopup=One filter per frame  IC=0  ICnum=0  ICden=0  roundingMode=Floor  overflowMode=off  ScaleValues=1  scaleValueFracLength=14  stageInFracLength=15  stageOutFracLength=15
  M : cdsSWD1/Subsystem
  POS_H1 : dsparch4/Digital Filter  DialogController=dspDDGCreate  DialogControllerArgs=DataTag82  TypePopup=IIR (poles & zeros)  IIRFiltStruct=Direct form II transposed  AllPoleFiltStruct=Direct form  FIRFiltStruct=Direct form  CoeffSource=Specify via dialog  NumCoeffs=[1 2]  DenCoeffs=[1 0.1]  BiQuadCoeffs=[1 0.3 0.4 1 0.1 0.2]  LatticeCoeffs=[0.2 0.4]  denIgnore=on  FiltPerSampPopup=One filter per frame  IC=0  ICnum=0  ICden=0  roundingMode=Floor  overflowMode=off  ScaleValues=1  scaleValueFracLength=14  stageInFracLength=15  stageOutFracLength=15
  POS_H2 : dsparch4/Digital Filter  DialogController=dspDDGCreate  DialogControllerArgs=DataTag83  TypePopup=IIR (poles & zeros)  IIRFiltStruct=Direct form II transposed  AllPoleFiltStruct=Direct form  FIRFiltStruct=Direct form  CoeffSource=Specify via dialog  NumCoeffs=[1 2]  DenCoeffs=[1 0.1]  BiQuadCoeffs=[1 0.3 0.4 1 0.1 0.2]  LatticeCoeffs=[0.2 0.4]  denIgnore=on  FiltPerSampPopup=One filter per frame  IC=0  ICnum=0  ICden=0  roundingMode=Floor  overflowMode=off  ScaleValues=1  scaleValueFracLength=14  stageInFracLength=15  stageOutFracLength=15
  POS_H3 : dsparch4/Digital Filter  DialogController=dspDDGCreate  DialogControllerArgs=DataTag84  TypePopup=IIR (poles & zeros)  IIRFiltStruct=Direct form II transposed  AllPoleFiltStruct=Direct form  FIRFiltStruct=Direct form  CoeffSource=Specify via dialog  NumCoeffs=[1 2]  DenCoeffs=[1 0.1]  BiQuadCoeffs=[1 0.3 0.4 1 0.1 0.2]  LatticeCoeffs=[0.2 0.4]  denIgnore=on  FiltPerSampPopup=One filter per frame  IC=0  ICnum=0  ICden=0  roundingMode=Floor  overflowMode=off  ScaleValues=1  scaleValueFracLength=14  stageInFracLength=15  stageOutFracLength=15
  POS_H4 : dsparch4/Digital Filter  DialogController=dspDDGCreate  DialogControllerArgs=DataTag85  TypePopup=IIR (poles & zeros)  IIRFiltStruct=Direct form II transposed  AllPoleFiltStruct=Direct form  FIRFiltStruct=Direct form  CoeffSource=Specify via dialog  NumCoeffs=[1 2]  DenCoeffs=[1 0.1]  BiQuadCoeffs=[1 0.3 0.4 1 0.1 0.2]  LatticeCoeffs=[0.2 0.4]  denIgnore=on  FiltPerSampPopup=One filter per frame  IC=0  ICnum=0  ICden=0  roundingMode=Floor  overflowMode=off  ScaleValues=1  scaleValueFracLength=14  stageInFracLength=15  stageOutFracLength=15
  POS_V1 : dsparch4/Digital Filter  DialogController=dspDDGCreate  DialogControllerArgs=DataTag86  TypePopup=IIR (poles & zeros)  IIRFiltStruct=Direct form II transposed  AllPoleFiltStruct=Direct form  FIRFiltStruct=Direct form  CoeffSource=Specify via dialog  NumCoeffs=[1 2]  DenCoeffs=[1 0.1]  BiQuadCoeffs=[1 0.3 0.4 1 0.1 0.2]  LatticeCoeffs=[0.2 0.4]  denIgnore=on  FiltPerSampPopup=One filter per frame  IC=0  ICnum=0  ICden=0  roundingMode=Floor  overflowMode=off  ScaleValues=1  scaleValueFracLength=14  stageInFracLength=15  stageOutFracLength=15
  POS_V2 : dsparch4/Digital Filter  DialogController=dspDDGCreate  DialogControllerArgs=DataTag87  TypePopup=IIR (poles & zeros)  IIRFiltStruct=Direct form II transposed  AllPoleFiltStruct=Direct form  FIRFiltStruct=Direct form  CoeffSource=Specify via dialog  NumCoeffs=[1 2]  DenCoeffs=[1 0.1]  BiQuadCoeffs=[1 0.3 0.4 1 0.1 0.2]  LatticeCoeffs=[0.2 0.4]  denIgnore=on  FiltPerSampPopup=One filter per frame  IC=0  ICnum=0  ICden=0  roundingMode=Floor  overflowMode=off  ScaleValues=1  scaleValueFracLength=14  stageInFracLength=15  stageOutFracLength=15
  POS_V3 : dsparch4/Digital Filter  DialogController=dspDDGCreate  DialogControllerArgs=DataTag88  TypePopup=IIR (poles & zeros)  IIRFiltStruct=Direct form II transposed  AllPoleFiltStruct=Direct form  FIRFiltStruct=Direct form  CoeffSource=Specify via dialog  NumCoeffs=[1 2]  DenCoeffs=[1 0.1]  BiQuadCoeffs=[1 0.3 0.4 1 0.1 0.2]  LatticeCoeffs=[0.2 0.4]  denIgnore=on  FiltPerSampPopup=One filter per frame  IC=0  ICnum=0  ICden=0  roundingMode=Floor  overflowMode=off  ScaleValues=1  scaleValueFracLength=14  stageInFracLength=15  stageOutFracLength=15
  POS_V4 : dsparch4/Digital Filter  DialogController=dspDDGCreate  DialogControllerArgs=DataTag89  TypePopup=IIR (poles & zeros)  IIRFiltStruct=Direct form II transposed  AllPoleFiltStruct=Direct form  FIRFiltStruct=Direct form  CoeffSource=Specify via dialog  NumCoeffs=[1 2]  DenCoeffs=[1 0.1]  BiQuadCoeffs=[1 0.3 0.4 1 0.1 0.2]  LatticeCoeffs=[0.2 0.4]  denIgnore=on  FiltPerSampPopup=One filter per frame  IC=0  ICnum=0  ICden=0  roundingMode=Floor  overflowMode=off  ScaleValues=1  scaleValueFracLength=14  stageInFracLength=15  stageOutFracLength=15
  STSX : dsparch4/Digital Filter  DialogController=dspDDGCreate  DialogControllerArgs=DataTag90  TypePopup=IIR (poles & zeros)  IIRFiltStruct=Direct form II transposed  AllPoleFiltStruct=Direct form  FIRFiltStruct=Direct form  CoeffSource=Specify via dialog  NumCoeffs=[1 2]  DenCoeffs=[1 0.1]  BiQuadCoeffs=[1 0.3 0.4 1 0.1 0.2]  LatticeCoeffs=[0.2 0.4]  denIgnore=on  FiltPerSampPopup=One filter per frame  IC=0  ICnum=0  ICden=0  roundingMode=Floor  overflowMode=off  ScaleValues=1  scaleValueFracLength=14  stageInFracLength=15  stageOutFracLength=15
  STSY : dsparch4/Digital Filter  DialogController=dspDDGCreate  DialogControllerArgs=DataTag91  TypePopup=IIR (poles & zeros)  IIRFiltStruct=Direct form II transposed  AllPoleFiltStruct=Direct form  FIRFiltStruct=Direct form  CoeffSource=Specify via dialog  NumCoeffs=[1 2]  DenCoeffs=[1 0.1]  BiQuadCoeffs=[1 0.3 0.4 1 0.1 0.2]  LatticeCoeffs=[0.2 0.4]  denIgnore=on  FiltPerSampPopup=One filter per frame  IC=0  ICnum=0  ICden=0  roundingMode=Floor  overflowMode=off  ScaleValues=1  scaleValueFracLength=14  stageInFracLength=15  stageOutFracLength=15
  STSZ : dsparch4/Digital Filter  DialogController=dspDDGCreate  DialogControllerArgs=DataTag92  TypePopup=IIR (poles & zeros)  IIRFiltStruct=Direct form II transposed  AllPoleFiltStruct=Direct form  FIRFiltStruct=Direct form  CoeffSource=Specify via dialog  NumCoeffs=[1 2]  DenCoeffs=[1 0.1]  BiQuadCoeffs=[1 0.3 0.4 1 0.1 0.2]  LatticeCoeffs=[0.2 0.4]  denIgnore=on  FiltPerSampPopup=One filter per frame  IC=0  ICnum=0  ICden=0  roundingMode=Floor  overflowMode=off  ScaleValues=1  scaleValueFracLength=14  stageInFracLength=15  stageOutFracLength=15
  wires:
  In1/1 -> STSX/1, M/1
  In2/1 -> STSY/1, M/3
  In3/1 -> STSZ/1, M/5
  In4/1 -> POS_V1/1, M/7
  STSX/1 -> M/2
  STSY/1 -> M/4
  STSZ/1 -> M/6
  POS_V1/1 -> M/8
  In5/1 -> POS_V2/1, M/9
  In6/1 -> POS_V3/1, M/11
  In7/1 -> POS_V4/1, M/13
  In8/1 -> POS_H1/1, M/15
  In9/1 -> POS_H2/1, M/17
  In10/1 -> POS_H3/1, M/19
  In11/1 -> POS_H4/1, M/21
  In12/1 -> GEO_V1/1, M/23
  In13/1 -> GEO_V2/1, M/25
  In14/1 -> GEO_V3/1, M/27
  In15/1 -> GEO_V4/1, M/29
  In16/1 -> GEO_H1/1, M/31
  In17/1 -> GEO_H2/1, M/33
  In18/1 -> GEO_H3/1, M/35
  In19/1 -> GEO_H4/1, M/37
  POS_V2/1 -> M/10
  POS_V3/1 -> M/12
  POS_V4/1 -> M/14
  POS_H1/1 -> M/16
  POS_H2/1 -> M/18
  POS_H3/1 -> M/20
  POS_H4/1 -> M/22
  GEO_V1/1 -> M/24
  GEO_V2/1 -> M/26
  GEO_V3/1 -> M/28
  GEO_V4/1 -> M/30
  GEO_H1/1 -> M/32
  GEO_H2/1 -> M/34
  GEO_H3/1 -> M/36
  GEO_H4/1 -> M/38
